simulink model "brain"  (Simulink 7.5)
settings: Solver=FixedStepDiscrete  StartTime=0.0  StopTime=inf  FixedStep=0.2  RelTol=1e-3
values from neighbouring files (symbols this model uses):
  Buoy1_Hue = 0.4    [brainconstants.m]    (also in brainconstants_David.m = 30)
  Buoy1_Saturation = 1.0    (= 1)    [brainconstants.m]    (also in brainconstants_David.m)
  Buoy1_Value = 0.45    [brainconstants.m]    (also in brainconstants_David.m)
  Buoy2_Hue = 0.0    (= 0)    [brainconstants.m]    (also in brainconstants_David.m = 80)
  Buoy2_Saturation = 1.0    (= 1)    [brainconstants.m]    (also in brainconstants_David.m)
  Buoy2_Value = 0.75    [brainconstants.m]    (also in brainconstants_David.m)
  Buoy_Max_Eccentricity = 0.7    [brainconstants.m]    (also in brainconstants_David.m = 1.2)
  Buoy_Max_Extent = 0.9    [brainconstants.m]    (also in brainconstants_David.m)
  Buoy_Min_Eccentricity = 0    [brainconstants.m]    (also in brainconstants_David.m)
  Buoy_Min_Extent = 0.7    [brainconstants.m]    (also in brainconstants_David.m = 0.1)
  Buoy_Strafe = 40    [brainconstants.m]    (also in brainconstants_David.m)
  Cam_Down_Strafe_XPos_Kd = 0.0    (= 0)    [brainconstants.m]    (also in brainconstants_David.m)
  Cam_Down_Strafe_XPos_Ki = 0.0    (= 0)    [brainconstants.m]    (also in brainconstants_David.m)
  Cam_Down_Strafe_XPos_Kp = -1.0    (= -1)    [brainconstants.m]    (also in brainconstants_David.m)
  Cam_Down_Yaw_XPos_Kd = 0.0    (= 0)    [brainconstants.m]    (also in brainconstants_David.m)
  Cam_Down_Yaw_XPos_Ki = 0.0    (= 0)    [brainconstants.m]    (also in brainconstants_David.m)
  Cam_Down_Yaw_XPos_Kp = 0.6    [brainconstants.m]    (also in brainconstants_David.m)
  Cam_Down_YPos_Kd = 0.0    (= 0)    [brainconstants.m]    (also in brainconstants_David.m)
  Cam_Down_YPos_Ki = 0.0    (= 0)    [brainconstants.m]    (also in brainconstants_David.m)
  Cam_Down_YPos_Kp = 0.75    [brainconstants.m]    (also in brainconstants_David.m)
  Cam_Forward_XPosition_Kd = 0.0    (= 0)    [brainconstants.m]    (also in brainconstants_David.m)
  Cam_Forward_XPosition_Ki = 0.0    (= 0)    [brainconstants.m]    (also in brainconstants_David.m)
  Cam_Forward_XPosition_Kp = 0.07    [brainconstants.m]    (also in brainconstants_David.m)
  Cam_Forward_YPosition_Kd = 0.0    (= 0)    [brainconstants.m]    (also in brainconstants_David.m)
  Cam_Forward_YPosition_Ki = 0.0    (= 0)    [brainconstants.m]    (also in brainconstants_David.m)
  Cam_Forward_YPosition_Kp = 0.8    [brainconstants.m]    (also in brainconstants_David.m)
  Depth_Kd = 0.0    (= 0)    [brainconstants.m]    (also in brainconstants_David.m)
  Depth_Ki = 0.0    (= 0)    [brainconstants.m]    (also in brainconstants_David.m)
  Depth_Kp = 75    [brainconstants.m]    (also in brainconstants_David.m)
  Heading_Forward_Velocity = 30    [brainconstants.m]    (also in brainconstants_David.m)
  Heading_Kd = 0.4    [brainconstants.m]    (also in brainconstants_David.m)
  Heading_Ki = 0.0    (= 0)    [brainconstants.m]    (also in brainconstants_David.m)
  Heading_Kp = 0.65    [brainconstants.m]    (also in brainconstants_David.m)
  Hedge_Hue = .4    (= 0.4)    [brainconstants.m]    (also in brainconstants_David.m)
  Hedge_Saturation = 1    [brainconstants.m]    (also in brainconstants_David.m)
  Hedge_Value = .75    (= 0.75)    [brainconstants.m]    (also in brainconstants_David.m)
  Iter_Segment_Thresh = 60    [brainconstants.m]    (also in brainconstants_David.m)
  MissionPlan = [1 1 1 1 1 1 1 1 1 1 1 1 1 0 0 0 0 0 0 0]    [brainconstants.m]    (also in brainconstants_David.m)
  Track_Desired_Depth = 8    [brainconstants.m]    (also in brainconstants_David.m)
  Track_HueHigher = 0.75    [brainconstants.m]    (also in brainconstants_David.m)
  Track_HueLower = 0.4    [brainconstants.m]    (also in brainconstants_David.m)
  Track_Min_Eccentricity = 0.9    [brainconstants.m]    (also in brainconstants_David.m)
  Track_Saturation = 0.75    [brainconstants.m]    (also in brainconstants_David.m)
  Vision_Forward_Velocity = 15    [brainconstants.m]    (also in brainconstants_David.m)
undefined symbols (not defined in the file or in its folder): DiscIntNeverNeededParam, gray, Rec, SDTV, strel, YawRate_Kd, YawRate_Ki, YawRate_Kp
libraries: vipconversions x32, simulink x26, vipgeotforms x9, vipstatistics x9, viptextngfix x7, vipmorphops x6, viptransforms x4, vipsnks x3, vipsrcs x1
(part 4 of 6)

== stateflow chart StateFlow Functions ==
  settings: updateMethod=DISCRETE  sampleTime=0.20
  state StateFlowFunctions [parallel]
    settings: executionOrder=3
    state NotRunning
      entry:
      Left = 0;
      Right = 0;
      Vertical = 0;
      Strafe = 0;
      State = -2;
    state ControlledRC
      entry:
      State = -1;
      exit:
      Left = 0;
      Right = 0;
      Strafe = 0;
      state Compass
        du:
        Vertical = MaintainDepth(CurrentDepth,RC_Depth);
        [Left,Right] = MaintainHeading(RC_Heading,CurrentHeading,RC_ForwardVelocity);
        Strafe = RC_Strafe;
      state IMU
        du:
        Vertical = MaintainDepth(CurrentDepth,RC_Depth);
        [Left, Right,Strafe] = GoStraight(YawRate,PitchAccelB,RC_ForwardVelocity);
      (default) -> Compass
      Compass -> IMU : [RC_Source > 0.5]
      IMU -> Compass : [RC_Source < 0.5]
    state Finish
      entry:
      State = 6;
      Left = 0;
      Right = 0;
      Vertical = 0;
      Strafe = 0;
    state [ChangetoLeft,ChangetoRight] = MaintainHeading(DesiredHeading1, CurrentHeading1, ForwardVelocity1) [function]
    state Buoys
      state RGBout = ShowSegmentedImage(LabMatrix,Ref_Colors) [function]
      state [LabelMatrix,num_colors,Ref_Colors] = IterativeSegmentation(H,S,V) [function]
      state BuoyDone
        en:
        Done = 1;
        Left = 0;
        Right = 0;
        Strafe = 0;
      state FindBuoys
        entry:
        Obstacle = 0;
        OldObstacle = 0;
        CameraPosition = 0;
        BuoyCount = 0;
        DesiredDepth = GetDesiredDepth();
        du:
        [LabelMatrix,num_colors,ref_colors] = IterativeSegmentation(H,S,V);
        RGBout = ShowSegmentedImage(LabelMatrix,ref_colors);
        [Obstacle, RGBout] = LookforBuoys(LabelMatrix,num_colors,RGBout);
        [BuoyCount] = countimages(Obstacle, OldObstacle, BuoyCount);
        Forward = GetBuoyForwardVelocity();
        [Left, Right] = MaintainHeading(DesiredHeading,CurrentHeading,Forward) ;
        [Vertical] = MaintainDepth(CurrentDepth,DesiredDepth);
        OldObstacle = Obstacle;
        exit:
        [BuoyBlobs, num_blobs] = GetBuoyColors(LabelMatrix,ref_colors,num_colors);
        state [Image,RGBout1] = LookforBuoys(LabMatrix,num_colors,RGBin) [function]
        state [L2RBlobs,num_blobs] = GetBuoyColors(LabelMatrix,ref_colors,num_colors) [function]
      state ForwardVel = GetBuoyForwardVelocity [function]
      state ApproachBuoys
        en:
        countarea = 0;
        count2ndarea = 0;
        TurnDirection = 0;
        state ApproachFirstBuoy
          entry:
          [BuoyHue,BuoySaturation,BuoyValue] = GetFirstBuoyStats();
          [FirstDir,SecondDir] = WhichBuoysToApproach(BuoyBlobs,num_blobs);
          du:
          [LabelMatrix,num_colors,ref_colors] = IterativeSegmentation(H,S,V);
          [Area, Right,Left, Vertical, BuoyCentroidX, BuoyCentroidY,BWout] = Buoy(LabelMatrix,ref_colors,num_colors,BuoyHue,BuoySaturation,BuoyValue);
          countarea = countareas(Area, countarea);
          RGBout = ShowSegmentedImage(LabelMatrix,ref_colors);
          state [B_H,B_S,B_V] = GetFirstBuoyStats [function]
          state [FirstD,SecondD] = WhichBuoysToApproach(buoys,num_blobs) [function]
        state [BuoyArea,ChangetoRight,ChangetoLeft,ChangetoVert,CentroidY,CentroidX,BWout1] = Buoy(LabMatrix,Ref_Colors,Num_Colors,B_Hue,B_Sat,B_Value) [function]
        state FindSecondBuoy
          en:
          TurnDirection = -1;
          DesiredHeading = Turn45Degrees(CurrentHeading,TurnDirection);
          DesiredDepth = CurrentDepth;
          [BuoyHue,BuoySaturation,BuoyValue] = GetSecondBuoyStats();
          Image = 0;
          du:
          [Left,Right] = MaintainHeading(DesiredHeading,CurrentHeading,0);
          Vertical = MaintainDepth(CurrentDepth,DesiredDepth);
          Strafe = GetStrafe();
          Strafe = TurnDirection * Strafe;
          [LabelMatrix,num_colors,ref_colors] = IterativeSegmentation(H,S,V);
          [Image, BWout] = SecondBuoy(LabelMatrix,ref_colors,num_colors,BuoyHue,BuoySaturation,BuoyValue);
          RGBout = ShowSegmentedImage(LabelMatrix,ref_colors);
          state [B_H,B_S,B_V] = GetSecondBuoyStats [function]
          state [Image,BWout1] = SecondBuoy(LabMatrix,Ref_Colors,Num_Colors,B_Hue,B_Sat,B_Value) [function]
          state Strafe1 = GetStrafe [function]
        state ApproachSecondBuoy
          entry:
          Strafe = 0;
          du:
          [LabelMatrix,num_colors,ref_colors] = IterativeSegmentation(H,S,V);
          [Area, Right,Left, Vertical, BuoyCentroidX, BuoyCentroidY,BWout] = Buoy(LabelMatrix,ref_colors,num_colors,BuoyHue,BuoySaturation,BuoyValue);
          count2ndarea = countareas(Area, count2ndarea);
          RGBout = ShowSegmentedImage(LabelMatrix,ref_colors);
        (default) -> ApproachFirstBuoy
        ApproachFirstBuoy -> FindSecondBuoy : [countarea>2]
        FindSecondBuoy -> ApproachSecondBuoy : [Image == 1]
      (default) -> FindBuoys
      FindBuoys -> ApproachBuoys : [BuoyCount > 2]
      ApproachBuoys -> BuoyDone : [count2ndarea > 2 || TurnDirection <= -999]
    state ValidationGate
      entry:
      Obstacle = 0;
      OldObstacle = 0;
      count = 0;
      TrackCount = 0;
      CameraPosition = 2;
      state GoThoughGate
        du:
        [Obstacle,BWout] = LookforTrack(H,S);
        [TrackCount] = countimages(Obstacle, OldObstacle, count);
        Forward = GetValidationGateForwardVelocity();
        [Left, Right] = MaintainHeading(DesiredHeading,CurrentHeading,Forward) ;
        [Vertical] = MaintainDepth(CurrentDepth,DesiredDepth);
        OldObstacle = Obstacle;
        count = TrackCount;
      state GateDone
        en:
        Done = 1;
      state [Image,BWout1] = LookforTrack(H,S) [function]
      state ForwardVel=GetValidationGateForwardVelocity [function]
      (default) -> GoThoughGate
      GoThoughGate -> GateDone : [TrackCount > 2]
    state ChangetoVertical = MaintainDepth(CurrentDepth1, DesiredDepth1) [function]
    state Start
      entry:
      OldHeading = 0;
      DesiredHeadingCount = 0;
      BuoyCentroidX = 0;
      BuoyCentroidY = 0;
      CameraPosition = 2;
      Left = 0;
      Right = 0;
      Vertical = 0;
      Strafe = 0;
      state GetHeadings
        du:
        DesiredHeadingCount = InitialHeadingCount(CurrentHeading,OldHeading,DesiredHeadingCount);
        OldHeading = CurrentHeading;
        DesiredDepth = GetDesiredDepth();
        exit:
        DesiredHeading = CurrentHeading;
      state StartFinished
        en:
        Done = 1;
      GetHeadings -> StartFinished : [DesiredHeadingCount >=3]
      (default) -> GetHeadings
    state GetInCorrectState
    state DesiredDepth = GetDesiredDepth [function]
    state FollowOnePath
      entry:
      DesiredDepth = GetDesiredDepth();
      DesiredHeading = CurrentHeading;
      CameraPosition = 2;
      Obstacle = 0;
      HSVImage = MakeHSVImage(H,S,V);
      state OnePath
        state Done
          en:
          Left = 0;
          Right = 0;
          Strafe = 0;
          DesiredHeading = CurrentHeading + HeadingAlongPath;
          Done = 1;
        state PositionOver
          en:
          Error = 500;
          du:
          BWout = HSVSegmentation(H,S);
          [Left,Right,Forward,ErrorX,ErrorY] = CamDown_CenterOver_Yaw(BWout);
          Vertical = MaintainDepth(CurrentDepth,DesiredDepth);
          Left = Left + Forward;
          Right = Right + Forward;
          Error = CalcError(ErrorX,ErrorY);
        state AlignWithPath
          entry:
          HeadingAlongPath = 10;
          Left = 0;
          Right = 0;
          Strafe = 0;
          du:
          [BWout] = HSVSegmentation(H,S);
          [HeadingAlongPath,BWout] = GetHeadings(BWout);
          [Left,Right,Forward,ErrorY,ErrorX] = CamDown_CenterOver_Yaw(BWout);
          Vertical = MaintainDepth(CurrentDepth,DesiredDepth);
          Strafe = Align(HeadingAlongPath);
          state Strafe = Align(HeadingAlong) [function]
          state [HeadingAlongPath1,BWout1] = GetHeadings(BW) [function]
        state BW1 = HSVSegmentation(H,S) [function]
        state [Strafe1,Forward1,ErrorX1,ErrorY1,BWout1] = CenterOver_Strafe(BW) [function]
        state [Left1,Right1,Forward1,ErrorY1,ErrorX1] = CamDown_CenterOver_Yaw(BW) [function]
        PositionOver -> AlignWithPath : [Error < 10]
        AlignWithPath -> StateFlowFunctions.FollowOnePath.OnePath.Done : [abs(HeadingAlongPath) <= 4]
        (default) -> PositionOver
      state RecognizePath
        du:
        [Obstacle,BWout] = LookforTrack(H,S);
        state TurnRight
          du:
          DesiredHeading = CurrentHeading + 15;
          [Left,Right] = MaintainHeading(DesiredHeading,CurrentHeading,0);
          [Vertical] = MaintainDepth(CurrentDepth,DesiredDepth);
        state TurnLeft
          du:
          DesiredHeading = CurrentHeading - 15;
          [Left,Right] = MaintainHeading(DesiredHeading,CurrentHeading,0);
          [Vertical] = MaintainDepth(CurrentDepth,DesiredDepth);
        state [Image,BWout1] = LookforTrack(H,S) [function]
        (default) -> TurnLeft
        TurnLeft -> TurnRight : after(1,sec)
        TurnRight -> TurnLeft : after(1,sec)
      state HSVImage1 = MakeHSVImage(H1,S1,V1) [function]
      (default) -> RecognizePath
      RecognizePath -> OnePath : [Obstacle == 1]
    state JumpHedge
      entry:
      Area = 1000;
      Left = 0;
      Right = 0;
      Strafe = 0;
      Done = 0;
      Image = 0;
      state ApproachHedge
        du:
        [LabelMatrix,num_colors,ref_colors] = IterativeSegmentation(H,S,V);
        BWout = IndividualSegmentation(LabelMatrix,ref_colors,num_colors,H_Hue,H_Sat,H_Value);
        [Left,Right,Vertical,BWout] = CameraForward_CenterOnBlobYaw(BWout,Forward);
        Area = GetArea(BWout);
        RGBout = ShowSegmentedImage(LabelMatrix,ref_colors);
        state AreaBiggestBlob = GetArea(BW) [function]
      state IncreaseAxisRatio
        exit:
        Strafe = 0;
        Left = 0;
        Right = 0;
        state Move
          du:
          [LabelMatrix,num_colors,ref_colors] = IterativeSegmentation(H,S,V);
          BWout = IndividualSegmentation(LabelMatrix,ref_colors,num_colors,H_Hue,H_Sat,H_Value);
          [Right,Left,Vertical] = CameraForward_CenterOnBlobYaw(BWout,0);
          Strafe = 40*StrafeDir;
          RGBout = ShowSegmentedImage(LabelMatrix,ref_colors);
          exit:
          Strafe = 0;
          Left = 0;
          Right = 0;
        state CheckAxisRatio
          en:
          NewAxisRatio = GetAxisRatio(BWout);
        (default) -> StateFlowFunctions.JumpHedge.IncreaseAxisRatio.Move
        StateFlowFunctions.JumpHedge.IncreaseAxisRatio.Move -> CheckAxisRatio : after(1,sec)
        CheckAxisRatio -> StateFlowFunctions.JumpHedge.IncreaseAxisRatio.Move
      state GetInitialDirection
        state GetMajorAxis
          entry:
          MoveOn = 0;
          OldAxisRatio = 0.5;
          StrafeDir = 1;
          [LabelMatrix,num_colors,ref_colors] = IterativeSegmentation(H,S,V);
          BWout = IndividualSegmentation(LabelMatrix,ref_colors,num_colors,H_Hue,H_Sat,H_Value);
          OldAxisRatio = GetAxisRatio(BWout);
          RGBout = ShowSegmentedImage(LabelMatrix,ref_colors);
        state Move
          du:
          [LabelMatrix,num_colors,ref_colors] = IterativeSegmentation(H,S,V);
          BWout = IndividualSegmentation(LabelMatrix,ref_colors,num_colors,H_Hue,H_Sat,H_Value);
          [Right,Left,Vertical] = CameraForward_CenterOnBlobYaw(BWout,0);
          Strafe = 40*StrafeDir;
          RGBout = ShowSegmentedImage(LabelMatrix,ref_colors);
          exit:
          Strafe = 0;
        state CompareAxisRatio
          entry:
          [LabelMatrix,num_colors,ref_colors] = IterativeSegmentation(H,S,V);
          BWout = IndividualSegmentation(LabelMatrix,ref_colors,num_colors,H_Hue,H_Sat,H_Value);
          NewAxisRatio = GetAxisRatio(BWout);
          AxisDifference = NewAxisRatio - OldAxisRatio;
          StrafeDir = GetStrafeDirection(AxisDifference);
          MoveOn = 1;
          RGBout = ShowSegmentedImage(LabelMatrix,ref_colors);
        (default) -> GetMajorAxis
        StateFlowFunctions.JumpHedge.GetInitialDirection.Move -> CompareAxisRatio : after(2,sec)
        GetMajorAxis -> StateFlowFunctions.JumpHedge.GetInitialDirection.Move
      state RecognizeHedge
        en:
        [H_Hue,H_Sat,H_Value] = GetHedgeValues();
        Forward = GetForwardVelocity();
        du:
        [LabelMatrix,num_colors,ref_colors] = IterativeSegmentation(H,S,V);
        BWout = IndividualSegmentation(LabelMatrix,ref_colors,num_colors,H_Hue,H_Sat,H_Value);
        [Left,Right] = MaintainHeading(DesiredHeading,CurrentHeading,Forward);
        [Vertical] = MaintainDepth(CurrentDepth,DesiredDepth);
        [Image,BWout] = LookForHedge(BWout);
        RGBout = ShowSegmentedImage(LabelMatrix,ref_colors);
        state [Image1,BWout1] = LookForHedge(BW) [function]
        state [H_hue,H_sat,H_val] = GetHedgeValues [function]
      state BW = IndividualSegmentation(LabMatrix,Ref_Colors,Num_Colors,B_Hue,B_Sat,B_Value) [function]
      state GoThroughHedge
        en:
        DesiredHeading = CurrentHeading;
        DesiredDepth = CurrentDepth - 2;
        Strafe = 0;
        du:
        [LabelMatrix,num_colors,ref_colors] = IterativeSegmentation(H,S,V);
        BWout = IndividualSegmentation(LabelMatrix,ref_colors,num_colors,H_Hue,H_Sat,H_Value);
        [Left,Right] = MaintainHeading(DesiredHeading,CurrentHeading,Forward);
        [Vertical] = MaintainDepth(CurrentDepth,DesiredDepth);
        RGBout = ShowSegmentedImage(LabelMatrix,ref_colors);
      state RGBout = ShowSegmentedImage(LabMatrix,Ref_Colors) [function]
      state [LabelMatrix,num_colors,Ref_Colors] = IterativeSegmentation(H,S,V) [function]
      state Finished
        en:
        Left = 0;
        Right = 0;
        Strafe = 0;
        Done = 1;
      state [ChangetoLeft,ChangetoRight,ChangetoVert,BWout1] = CameraForward_CenterOnBlobYaw(BW,ForwardVelocity) [function]
      state AxisRatio = GetAxisRatio(BW) [function]
      state ForwardVel=GetForwardVelocity [function]
      GetInitialDirection -> ApproachHedge [order 1] : [OldAxisRatio > 1 || NewAxisRatio > 1]
      (default) -> RecognizeHedge
      RecognizeHedge -> GetInitialDirection : [Image == 1]
      IncreaseAxisRatio -> ApproachHedge : [NewAxisRatio > 1]
      GetInitialDirection -> IncreaseAxisRatio [order 2] : [MoveOn == 1]
      ApproachHedge -> GoThroughHedge : [Area > 4000]
      GoThroughHedge -> StateFlowFunctions.JumpHedge.Finished : after(5,sec)
    state DropMechanism
      en:
      Done = 1;
    state LocatePinger
      en:
      Done = 1;
      MoveOn = 0;
      OldDesiredHeading = DesiredHeading;
      exit:
      Left = 0;
      Right = 0;
      Vertical = 0;
      state Finished
        en:
        Done = changemeasure(DesiredHeading,OldDesiredHeading);
      state GetPingerHeading
        en:
        Left = 0;
        Right = 0;
        OldDesiredHeading = DesiredHeading;
        du:
        Vertical = MaintainDepth(CurrentDepth,DesiredDepth);
        state FirstDirections
          en:
          [Heading1, Heading2] = GetHeadings();
        state SecondDirections
          en:
          Left = 0;
          Right = 0;
          [Heading3,Heading4] = GetHeadings();
        state Turn30Degrees
          en:
          DesiredHeading = Turn30(CurrentHeading);
          du:
          [Left,Right] = MaintainHeading(DesiredHeading,CurrentDepth,0);
        state GetActualDirection
          en:
          DesiredHeading = ProperHeading(Heading1,Heading2,Heading3,Heading4);
        state GoToNext
          MoveOn = 1;
        state [Heading11,Heading22] = GetHeadings [function]
        FirstDirections -> Turn30Degrees
        Turn30Degrees -> SecondDirections : [abs(CurrentHeading-DesiredHeading) < 5]
        SecondDirections -> GetActualDirection
        GetActualDirection -> FirstDirections [order 1] : [DesiredHeading == -1]
        GetActualDirection -> GoToNext [order 2] : [DesiredHeading ~= -1]
        (default) -> FirstDirections
      state Move
        du:
        [Left,Right] = MaintainHeading(DesiredHeading,CurrentHeading,Forward);
        Vertical = MaintainDepth(CurrentDepth,DesiredDepth);
      GetPingerHeading -> StateFlowFunctions.LocatePinger.Finished : [MoveOn ~= 0]
      StateFlowFunctions.LocatePinger.Move -> GetPingerHeading : after(3,sec)
      StateFlowFunctions.LocatePinger.Finished -> StateFlowFunctions.LocatePinger.Move
      (default) -> GetPingerHeading
    state Breach
      en:
      Left = 0;
      Right = 0;
      Vertical = -127;
      Strafe = 0;
      exit:
      Vertical = 0;
      state GoUpNCheck
      state MakeSure
      state Done
        Done = 1;
      (default) -> GoUpNCheck
      GoUpNCheck -> MakeSure : [CurrentDepth < 0.5]
      MakeSure -> StateFlowFunctions.Breach.Done : after(3,sec)
    state [ChangetoLeft1,ChangetoRight1,Strafe1] = GoStraight(YawRate,ForwardVelocity1,Y_Accel) [function]
    StateFlowFunctions.Finish -> GetInCorrectState : [OperationalState ~= 9]
    (default) -> GetInCorrectState
    StateFlowFunctions.NotRunning -> GetInCorrectState : [OperationalState ~= -2]
    GetInCorrectState -> StateFlowFunctions.NotRunning [order 1] : [OperationalState == -2]
    GetInCorrectState -> StateFlowFunctions.ControlledRC [order 3] : [OperationalState == -1]
    StateFlowFunctions.ControlledRC -> GetInCorrectState : [OperationalState ~= -1]
    StateFlowFunctions.Start -> GetInCorrectState : [OperationalState ~= 1]
    GetInCorrectState -> StateFlowFunctions.Start [order 4] : [OperationalState == 1]
    GetInCorrectState -> StateFlowFunctions.ValidationGate [order 5] : [OperationalState == 2]
    StateFlowFunctions.ValidationGate -> GetInCorrectState : [OperationalState ~= 2]
    FollowOnePath -> GetInCorrectState : [OperationalState ~= 3]
    GetInCorrectState -> FollowOnePath [order 7] : [OperationalState == 3]
    Buoys -> GetInCorrectState : [OperationalState ~= 4]
    GetInCorrectState -> Buoys [order 8] : [OperationalState == 4]
    GetInCorrectState -> StateFlowFunctions.Finish [order 6] : [OperationalState == 9]
    GetInCorrectState -> JumpHedge [order 2] : [OperationalState == 5]
    JumpHedge -> GetInCorrectState : [OperationalState ~= 5]
    StateFlowFunctions.DropMechanism -> GetInCorrectState : [OperationalState ~= 6]
    GetInCorrectState -> StateFlowFunctions.DropMechanism [order 9] : [OperationalState == 6]
    GetInCorrectState -> StateFlowFunctions.LocatePinger [order 10] : [OperationalState == 7]
    StateFlowFunctions.LocatePinger -> GetInCorrectState : [OperationalState ~= 7]
    GetInCorrectState -> StateFlowFunctions.Breach [order 11] : [OperationalState == 8]
    StateFlowFunctions.Breach -> GetInCorrectState : [OperationalState ~=8]
  state StateManagement [parallel]
    settings: executionOrder=2
    state NotRunning
      en:
      Done = 0;
      du:
      OperationalState = -2;
    state Running
      state Autonomous
        state Buoy
          en:
          State = 4;
          Done = Perform(State);
          du:
          OperationalState = 4;
        state ValidationGate
          en:
          State = 2;
          Done = Perform(State);
          du:
          OperationalState = 2;
        state Finish
          en:
          State = 13;
          Done = Perform(State);
          du:
          OperationalState = 9;
        state FollowOnePath1
          en:
          State = 3;
          Done = Perform(State);
          du:
          OperationalState = 3;
        state ChooseState
          en:
          Done = 0;
        state FollowOnePath2
          en:
          State = 5;
          Done = Perform(State);
          du:
          OperationalState = 3;
        state Start
          en:
          State = 1;
          Done = Perform(State);
          du:
          OperationalState = 1;
        state Hedge1
          en:
          State = 6;
          Done = Perform(State);
          du:
          OperationalState = 5;
        state FollowOnePath3
          en:
          State = 7;
          Done = Perform(State);
          du:
          OperationalState = 3;
        state DropMechanism
          en:
          State = 8;
          Done = Perform(State);
          du:
          OperationalState = 6;
        state FollowOnePath4
          en:
          State = 9;
          Done = Perform(State);
          du:
          OperationalState = 3;
        state Hedge2
          en:
          State = 10;
          Done = Perform(State);
          du:
          OperationalState = 5;
        state LocatePinger
          en:
          State = 11;
          Done = Perform(State);
          du:
          OperationalState = 7;
        state Breach
          en:
          State = 12;
          Done = Perform(State);
          du:
          OperationalState = 8;
        state Done1 = Perform(State1) [function]
        FollowOnePath1 -> ChooseState [order 2] : [DesiredState ~= 3 && DesiredState ~= 0]
        ChooseState -> FollowOnePath1 [order 6] : [DesiredState == 3]
        StateManagement.Running.Autonomous.ValidationGate -> ChooseState [order 1] : [DesiredState ~= 2 && DesiredState ~= 0]
        ChooseState -> StateManagement.Running.Autonomous.ValidationGate [order 3] : [DesiredState == 2]
        FollowOnePath2 -> ChooseState [order 1] : [DesiredState ~= 5 && DesiredState ~= 0]
        ChooseState -> FollowOnePath2 [order 7] : [DesiredState == 5]
        FollowOnePath1 -> Buoy [order 1] : [Done ~= 0 && DesiredState == 0]
        Buoy -> FollowOnePath2 [order 1] : [Done ~= 0 && DesiredState == 0]
        StateManagement.Running.Autonomous.Breach -> StateManagement.Running.Autonomous.Finish [order 2] : [Done ~= 0 && DesiredState == 0]
        StateManagement.Running.Autonomous.Start -> StateManagement.Running.Autonomous.ValidationGate [order 1] : [Done ~= 0 && DesiredState == 0]
        StateManagement.Running.Autonomous.ValidationGate -> FollowOnePath1 [order 2] : [Done ~=0 && DesiredState == 0]
        (default) -> StateManagement.Running.Autonomous.Start
        ChooseState -> Buoy [order 4] : [DesiredState == 4]
        StateManagement.Running.Autonomous.Finish -> ChooseState : [DesiredState ~= 7 && DesiredState ~= 7]
        StateManagement.Running.Autonomous.Start -> ChooseState [order 2] : [DesiredState ~= 1 && DesiredState ~= 0]
        ChooseState -> StateManagement.Running.Autonomous.Start [order 1] : [DesiredState == 1 || DesiredState == 0]
        Buoy -> ChooseState [order 2] : [DesiredState ~= 4 && DesiredState ~= 0]
        FollowOnePath2 -> Hedge1 [order 2] : [Done ~= 0 && DesiredState == 0]
        Hedge1 -> ChooseState [order 1] : [DesiredState ~= 6 && DesiredState ~= 0]
        ChooseState -> Hedge1 [order 2] : [DesiredState == 6]
        Hedge1 -> FollowOnePath3 [order 2] : [Done ~= 0 && DesiredState == 0]
        FollowOnePath3 -> ChooseState [order 1] : [DesiredState ~= 7 && DesiredState ~= 0]
        ChooseState -> FollowOnePath3 [order 8] : [DesiredState == 7]
        FollowOnePath3 -> StateManagement.Running.Autonomous.DropMechanism [order 2] : [Done ~= 0 && DesiredState == 0]
        StateManagement.Running.Autonomous.DropMechanism -> ChooseState [order 1] : [DesiredState ~= 8 && DesiredState ~= 0]
        ChooseState -> StateManagement.Running.Autonomous.DropMechanism [order 9] : [DesiredState == 8]
        FollowOnePath4 -> ChooseState [order 1] : [DesiredState ~= 0 && DesiredState ~= 9]
        ChooseState -> FollowOnePath4 [order 10] : [DesiredState == 9]
        Hedge2 -> ChooseState [order 1] : [DesiredState ~= 0 && DesiredState ~= 10]
        ChooseState -> Hedge2 [order 11] : [DesiredState == 10]
        FollowOnePath4 -> Hedge2 [order 2] : [Done ~= 0 && DesiredState == 0]
        StateManagement.Running.Autonomous.LocatePinger -> ChooseState [order 1] : [DesiredState ~= 0 && DesiredState ~= 11]
        ChooseState -> StateManagement.Running.Autonomous.LocatePinger [order 5] : [DesiredState == 11]
        Hedge2 -> StateManagement.Running.Autonomous.LocatePinger [order 2] : [Done ~= 0 && DesiredState == 0]
        StateManagement.Running.Autonomous.DropMechanism -> FollowOnePath4 [order 2] : [Done ~= 0 && DesiredState == 0]
        StateManagement.Running.Autonomous.Breach -> ChooseState [order 1] : [DesiredState ~= 0 && DesiredState ~= 12]
        ChooseState -> StateManagement.Running.Autonomous.Breach [order 12] : [DesiredState == 12]
        StateManagement.Running.Autonomous.LocatePinger -> StateManagement.Running.Autonomous.Breach [order 2] : [Done ~= 0 && DesiredState == 0]
      state ControlledRC
        du:
        OperationalState = -1;
      StateManagement.Running.ControlledRC -> Autonomous : [RC == 0]
      Autonomous -> StateManagement.Running.ControlledRC : [RC == 1]
      (default) -> Autonomous
    Running -> StateManagement.NotRunning : [Status ~= 1]
    (default) -> StateManagement.NotRunning
    StateManagement.NotRunning -> Running : [Status == 1]
  state StateEstimator [parallel]
    du:
    Tare1 = Tare;
    settings: executionOrder=1
    state CalcTare
      en:
      TareDone = 0;
      state PerformTare
        en:
        DeltaT1 = CheckDeltaT(DeltaT);
        Yaw1 = CurrentHeading - TarYaw;
        YawRate1 = YawRate - TarYawRate;
        Pitch1 = PitchEuler - TarPitch;
        PitchRate1 = PitchRate - TarPitchRate;
        Roll1 = RollEuler - TarRoll;
        RollRate1 = RollRate - TarRollRate;
        YawRate_Model = AUV_Yaw_Model(Left,Right,OldYawRate,DeltaT1);
        YawRate_Out = combinevalues(YawRate_Model,YawRate1,0.7,0.48);
        OldYawRate = YawRate_Out;
        [Yaw_IMU, Pitch_IMU, Roll_IMU] = Integrate3(YawRate_Out,PitchRate1,RollRate1,OldYaw,OldPitch,OldRoll,DeltaT1);
        Yaw = Yaw_IMU;
        OldYaw = Yaw;
        Pitch = combinevalues(Pitch_IMU,Pitch1,0.75,1);
        OldPitch = Pitch;
        Roll = combinevalues(Roll_IMU,Roll1,0.75,1);
        [Yaw_IMU, Pitch_IMU, Roll_IMU] = Integrate3(YawRate,PitchRate,RollRate,OldYaw,OldPitch,OldRoll,DeltaT1);
        Yaw = combinevalues(Yaw_IMU,CurrentHeading,.75,1);
        OldYaw = Yaw;
        Pitch = combinevalues(Pitch_IMU,PitchEuler,.75,1);
        OldPitch = Pitch;
        Roll = combinevalues(Roll_IMU,RollEuler,.75,1);
        OldRoll = Roll;
        TRA = RollAccelB;
        TPA = PitchAccelB;
        TYA = YawAccelB;
      state Stop
        en:
        Left = 0;
        Right = 0;
        Strafe = 0;
        Vertical = 0;
        stepcount = 0;
        TarYaw = CurrentHeading;
        TarYawRate = YawRate;
        TarPitch = PitchEuler;
        TarPitchRate = PitchRate;
        TarRoll = RollEuler;
        TarRollRate = RollRate;
        OldYaw = 0;
        OldYawRate = 0;
        OldPitch = 0;
        OldRoll = 0;
        OldXVel = 0;
        OldYVel = 0;
        OldZVel = 0;
        OldX = 0;
        OldY = 0;
        OldZ = 0;
        du:
        stepcount = stepcount + 1;
      state Next
        en:
        TareDone = 1;
      (default) -> Stop
      Stop -> PerformTare : [stepcount >= 10]
      PerformTare -> Next
    state CalcIMUInfo
      du:
      DeltaT1 = CheckDeltaT(DeltaT);
      YawRate1 = YawRate - TarYawRate;
      Pitch1 = PitchEuler - TarPitch;
      PitchRate1 = PitchRate - TarPitchRate;
      Roll1 = RollEuler - TarRoll;
      RollRate1 = RollRate - TarRollRate;
      YawRate_Model = AUV_Yaw_Model(Left,Right,OldYawRate,DeltaT1);
      YawRate_Out = combinevalues(YawRate_Model,YawRate1,0.7,0.48);
      OldYawRate = YawRate_Out;
      PitchRate_Out = PitchRate1;
      RollRate_Out = RollRate1;
      [Yaw_IMU, Pitch_IMU, Roll_IMU] = Integrate3(YawRate_Out,PitchRate1,RollRate1,OldYaw,OldPitch,OldRoll,DeltaT1);
      Yaw = Yaw_IMU;
      OldYaw = Yaw;
      Pitch = combinevalues(Pitch_IMU,Pitch1,0.75,1);
      OldPitch = Pitch;
      Roll = combinevalues(Roll_IMU,Roll1,0.75,1);
      OldRoll = Roll;
      Roll_AccelB = (RollAccelB - TRA)/0.3048;
      Pitch_AccelB = (PitchAccelB - TPA)/0.3048;
      Yaw_AccelB = (YawAccelB - TYA)/0.3048;
      [Roll_Accel,Pitch_Accel,Yaw_Accel] = GoToEarthCFrame(Roll_AccelB,Pitch_AccelB,Yaw_AccelB,Yaw,Pitch,Roll);
      [XVel,YVel,ZVel] = Integrate3(Roll_Accel,Pitch_Accel,Yaw_Accel,OldXVel,OldYVel,OldZVel,DeltaT1);
      OldXVel = XVel;
      OldYVel = YVel;
      OldZVel = ZVel;
      [X,Y,Z] = Integrate3(XVel,YVel,ZVel,OldX,OldY,OldZ,DeltaT1);
    (default) -> CalcTare
    CalcIMUInfo -> CalcTare : [Tare1 > 0.5]
    CalcTare -> CalcIMUInfo : [TareDone > 0.5]
  data: CHeading function_input double; TurnD function_input double; DHeading function_output double; FirstD function_input double; SecondD function_input double; TurnD function_output double; B_H function_output double; B_S function_output double; B_V function_output double; LabMatrix function_input double; Ref_Colors function_input double; BuoyArea function_output double; ChangetoRight function_output double; ChangetoLeft function_output double; ChangetoVert function_output double; CentroidY function_output double; CentroidX function_output double; BWout1 function_output double; Num_Colors function_input double; B_Hue function_input double; B_Sat function_input double; B_Value function_input double; LabMatrix function_input double; num_colors function_input double; Image function_output double; RGBin function_input double; RGBout1 function_output double; Size function_input double; count1 function_input double; count2 function_output double; LabMatrix function_input double; Ref_Colors function_input double; RGBout function_output double; H function_input double; S function_input double; V function_input double; LabelMatrix function_output double; num_colors function_output double; Ref_Colors function_output double; LabelMatrix function_input double; ref_colors function_input double; num_colors function_input double; L2RBlobs function_output double; num_blobs function_output double; DesiredHeading1 function_input double; CurrentHeading1 function_input double; ChangetoLeft function_output double; ChangetoRight function_output double; ForwardVelocity1 function_input double; B_H function_output double; B_S function_output double; B_V function_output double; Image function_output double; LabMatrix function_input double; Ref_Colors function_input double; BWout1 function_output double; Num_Colors function_input double; B_Hue function_input double; B_Sat function_input double; B_Value function_input double; ForwardVel function_output double; buoys function_input double; num_blobs function_input double; FirstD function_output double; SecondD function_output double; Image1 function_input double; OldImage function_input double; count1 function_input double; count2 function_output double; Strafe1 function_output double; Image function_input double; OldImage function_input double; count1 function_input double; count2 function_output double; Image function_output double; H function_input double; S function_input double; BWout1 function_output double; ForwardVel function_output double; CurrentDepth1 function_input double; DesiredDepth1 function_input double; ChangetoVertical function_output double; CurrentHeading1 function_input double; DesiredHeadingCount1 function_output double; OldHeading1 function_input double; count1 function_input double; DesiredDepth function_output double; ErrorX1 function_input double; ErrorY1 function_input double; Error1 function_output double; HeadingAlong function_input double; Strafe function_output double; BW function_input double; HeadingAlongPath1 function_output double; BWout1 function_output double; H function_input double; BW1 function_output double; S function_input double; BW function_input double; Strafe1 function_output double; Forward1 function_output double; ErrorX1 function_output double; ErrorY1 function_output double; BWout1 function_output double; Image function_output double; H function_input double; S function_input double; BWout1 function_output double; H1 function_input double; S1 function_input double; V1 function_input double; HSVImage1 function_output double; AreaBiggestBlob function_output double; BW function_input double; AxisDif function_input double; StrafeDir1 function_output double; BW function_input double; Image1 function_output double; BWout1 function_output double; H_hue function_output double; H_sat function_output double; H_val function_output double; LabMatrix function_input double; Ref_Colors function_input double; Num_Colors function_input double; B_Hue function_input double; B_Sat function_input double; B_Value function_input double; BW function_output double; LabMatrix function_input double; Ref_Colors function_input double; RGBout function_output double; H function_input double; S function_input double; V function_input double; LabelMatrix function_output double; num_colors function_output double; Ref_Colors function_output double; ChangetoLeft function_output double; ChangetoRight function_output double; ChangetoVert function_output double; BW function_input double; ForwardVelocity function_input double; BWout1 function_output double; BW function_input double; AxisRatio function_output double; AxisDif function_input double; StrafeDirection function_input double; Strafeout function_output double; ForwardVel function_output double; CurrentDepth1 function_input double; Done1 function_output double; signal1 function_input double; DesiredHeading1 function_output double; DesiredHeading1 function_input double; OldDesiredHeading1 function_input double; finished function_output double; CurrentHeading1 function_input double; heading function_output double; Heading11 function_input double; Heading22 function_input double; Heading33 function_input double; Heading44 function_input double; heading function_output double; Heading11 function_output double; Heading22 function_output double; State1 function_input double; Done1 function_output double; BW function_input double; Left1 function_output double; Right1 function_output double; Forward1 function_output double; ErrorY1 function_output double; ErrorX1 function_output double; YawRate function_input double; ForwardVelocity1 function_input double; ChangetoLeft1 function_output double; ChangetoRight1 function_output double; Y_Accel function_input double; Strafe1 function_output double; r function_input double; yaw1 function_input double; value function_output double; deltaT function_input double; Yr function_input double; Pr function_input double; Rr function_input double; OY function_input double; OP function_input double; OR function_input double; Y1 function_output double; P1 function_output double; R1 function_output double; deltaT function_input double; delta function_input double; delta1 function_output double; RAccB function_input double; PAccB function_input double; YAccB function_input double; R_Acc function_output double; P_Acc function_output double; Y_Acc function_output double; y function_input double; p function_input double; r function_input double; r_m function_input double; r1 function_input double; r function_output double; e1 function_input double; e2 function_input double; L1 function_input double; R1 function_input double; r_0 function_input double; r function_output double; deltaT function_input double; Left output int8 size=1; CurrentDepth input double size=1; CurrentHeading input double size=1; Right output int8 size=1; Strafe output int8; Vertical output int8 size=1; DesiredDepth output double; count local double; Obstacle local boolean size=1; OldObstacle local boolean; DesiredHeading output double; Area local int32; countarea local double; CameraPosition output int8 size=1; H input single size=[120 160]; S input single size=[120 160]; V input single size=[120 160]; BuoyCentroidX output double; BuoyCentroidY output double; DesiredHeadingCount local double; OldHeading local double; TrackCount local double; BuoyCount local double; State output int8 size=1; Status input int8 size=1; DesiredState input int8; HSVImage local double size=[120 160 3]; HeadingAlongPath local double; Done local double; RC_Heading input double; RC_ForwardVelocity input double; RC_Strafe input double; RC_Depth input double; RC input boolean; Error local double; ErrorX local double; ErrorY local double; Forward local double; BWout output double size=[120 160]; OperationalState local int8; BuoyHue local double; BuoySaturation local double; BuoyValue local double; FirstDir local double; Image local double; LabelMatrix local double size=[120 160]; RGBout output double size=[120 160 3]; SecondDir local double; TurnDirection local double; count2ndarea local double; num_colors local double; ref_colors local double size=[50 3]; num_blobs local double; BuoyBlobs local double size=[50 4]; AxisDifference local double; H_Hue local double; H_Sat local double; H_Value local double; MoveOn local double; NewAxisRatio local double; OldAxisRatio local double; StrafeDir local double; Heading1 local double; Heading2 local double; Heading3 local double; Heading4 local double; OldDesiredHeading local double; YawRate input double; PitchRate input double; PitchAccelB input double; PitchEuler input double; RollRate input double; RollAccelB input double; RollEuler input double; YawAccelB input double; Tare input double; DeltaT input double; OldPitch local double; OldRoll local double; OldX local double; OldXVel local double; OldY local double; OldYVel local double; OldYaw local double; OldYawRate local double; OldZ local double; OldZVel local double; Pitch_IMU local double; Roll_IMU local double; TPA local double; TRA local double; TYA local double; YawRate_Model local double; Yaw_IMU local double; Tare1 local double; stepcount local double; Pitch output double; Roll output double; Yaw output double; X output double; Y output double; Z output double; XVel output double; YVel output double; ZVel output double; Pitch_Accel output double; Roll_Accel output double; Yaw_Accel output double; PitchRate_Out output double; RollRate_Out output double; YawRate_Out output double; RC_Source input double; DeltaT1 local double; Pitch1 local double; PitchRate1 local double; Roll1 local double; RollRate1 local double; TarPitch local double; TarPitchRate local double; TarRoll local double; TarRollRate local double; TarYaw local double; TarYawRate local double; Yaw1 local double; YawRate1 local double; Pitch_AccelB local double; Roll_AccelB local double; TareDone local double; Yaw_AccelB local double
  function DHeading = Turn45Degrees(CHeading,TurnD):
    | function DHeading = Turn45Degrees(CHeading,TurnD)
    | % This function changes the current heading by 45 degrees in the correct
    | % direction to see the next buoy
    | 
    | DHeading = CHeading + TurnD*45;
    | 
    | if(DHeading > 360)
    |     DHeading = DHeading - 360;
    | elseif(DHeading < 0)
    |     DHeading = DHeading + 360;
    | end
    | 
    | return
  function TurnD = GetDirectionToLook(FirstD,SecondD):
    | function TurnD = GetDirectionToLook(FirstD,SecondD)
    | % Determine which direction the AUV needs to turn to see the next buoy
    | % -1 is left, 1 is right, -999 is for a single buoy attempt
    | 
    | % FirstD, SecondD are 1,2,3 - left,middle,right
    | TurnD = SecondD - FirstD;
    | 
    | if(TurnD ~= 0)
    |     TurnD = TurnD / abs(TurnD);
    | else
    |     TurnD = -999;
    | end
    | 
    | return
  function count2 = countareas(Size, count1):
    | function count2 = countareas(Size, count1)
    | % This function acts to count the number of consecutive times a particular
    | % area is recognized by the recognition software
    | 
    | count2 = count1;
    | if(Size > 16000)
    |     count2 = count2 + 1;
    | else
    |     count2 = 0;
    | end
  function count2 = countimages(Image1, OldImage, count1):
    | function count2 = countimages(Image1, OldImage, count1)
    | % This function acts to count the number of consecutive times a particular
    | % image is recognized by the recognition software
    | 
    | count2 = count1;
    | if(Image1 == 1)
    |     count2 = count2 + 1;
    | else
    |     count2 = 0;
    | end
  function count2 = countimages(Image, OldImage, count1):
    | function count2 = countimages(Image, OldImage, count1)
    | % This function acts to count the number of consecutive times a particular
    | % image is recognized by the recognition software
    | 
    | count2 = count1;
    | if(Image ~= 0 && Image == OldImage)
    |     count2 = count2 + 1;
    | else
    |     count2 = 0;
    | end
  function DesiredHeadingCount1 = InitialHeadingCount(CurrentHeading1,OldHeading1,count1):
    | function DesiredHeadingCount1 = InitialHeadingCount(CurrentHeading1,OldHeading1,count1)
    | 
    | tolerance = 2;
    | 
    | if(CurrentHeading1 > OldHeading1 - tolerance && CurrentHeading1 < OldHeading1 + tolerance)
    |     count1 = count1 + 1;
    | else
    |     count1 = 0;
    | end
    | DesiredHeadingCount1 = count1;
  function Error1 = CalcError(ErrorX1,ErrorY1):
    | function Error1 = CalcError(ErrorX1,ErrorY1)
    | % This function calculates the error between the center of the screen and 
    | % the centroid of the orange/red blob
    | 
    | Error1 = abs(ErrorX1) + abs(ErrorY1);
    | 
    | return
  function StrafeDir1 = GetStrafeDirection(AxisDif):
    | function StrafeDir1 = GetStrafeDirection(AxisDif)
    | % This function determines the direction the AUV should be strafing based
    | % on the initial major axis length change when strafing right
    | 
    | if(AxisDif < 0)
    |     StrafeDir1 = -1;
    | else
    |     StrafeDir1 = 1;
    | end
    | 
    | % StrafeDir = -1 corresponds to strafing left
    | % StrafeDir = 1 corresponds to strafing right
    | 
    | return
  function Strafeout = CalcStrafe(AxisDif,StrafeDirection):
    | function Strafeout = CalcStrafe(AxisDif,StrafeDirection)
    | % This function determines the current command to the strafing thruster
    | 
    | Kp = 4;
    | 
    | Strafeout = Kp * AxisDif * StrafeDirection;
    | 
    | return
  function Done1 = BreachDone(CurrentDepth1):
    | function Done1 = BreachDone(CurrentDepth1)
    | % This function determines if the vehicle has breached
    | 
    | if(CurrentDepth1 < 0.5)
    |     Done1 = 1;
    | else
    |     Done1 = 0;
    | end
    | 
    | return
  function DesiredHeading1=CalcPingerDirection(signal1):
    | function DesiredHeading1=CalcPingerDirection(signal1)
    | % This function determines the direction to the pinger given a signal from
    | % it
    | 
    | DesiredHeading1 = 0;
    | 
    | return
  function finished = changemeasure(DesiredHeading1,OldDesiredHeading1):
    | function finished = changemeasure(DesiredHeading1,OldDesiredHeading1)
    | % This function determines if the heading changes a large enough amount to 
    | % imply that the auv is above the pinger
    | 
    | finished = 0;
    | 
    | heading_change = DesiredHeading1 - OldDesiredHeading1;
    | 
    | if(abs(heading_change) > 60)
    |     finished = 1;
    | end
    | 
    | return
  function heading = Turn30(CurrentHeading1):
    | function heading = Turn30(CurrentHeading1)
    | % This function determines the heading to turn 30 degrees to the right
    | 
    | heading = CurrentHeading1 + 30;
    | 
    | if(heading >= 360)
    |     heading = heading - 360;
    | end
    | 
    | return
  function heading = ProperHeading(Heading11,Heading22,Heading33,Heading44):
    | function heading = ProperHeading(Heading11,Heading22,Heading33,Heading44)
    | % This function finds the two headings that match, giving the actual
    | % heading to the pinger
    | 
    | differences = zeros(4,4);
    | 
    | Headings = zeros(1,4);
    | 
    | Headings(1) = Heading11;
    | Headings(2) = Heading22;
    | Headings(3) = Heading33;
    | Headings(4) = Heading44;
    | 
    | for i = 1:4
    |     for j = 1:4
    |         differences(i,j) = abs(Headings(i) - Headings(j));
    |     end
    | end
    | 
    | index = 1;
    | min_dif = 1000;
    | for i = 1:2
    |     for j = 3:4
    |         if(i ~= j)
    |             if(differences(i,j) < min_dif)
    |                 min_dif = differences(i,j);
    |                 index = i;
    |             end
    |         end
    |     end
    | end
    | 
    | if(min_dif < 5)
    |     heading = Headings(index);
    | else
    |     heading = -1;
    | end
    | 
    | return
  function value  = Integrate(r,yaw1,deltaT):
    | function value  = Integrate(r,yaw1,deltaT)
    | % This function performs simple integration
    | 
    | value = r*deltaT + yaw1;
    | 
    | return
  function [Y1,P1,R1] = Integrate3(Yr,Pr,Rr,OY,OP,OR,deltaT):
    | function [Y1,P1,R1] = Integrate3(Yr,Pr,Rr,OY,OP,OR,deltaT)
    | % This function calculates the euler angles using an IMU approach
    | 
    | Y1 = Yr*deltaT + OY;
    | P1 = Pr*deltaT + OP;
    | R1 = Rr*deltaT + OR;
    | 
    | return
  function delta1 = CheckDeltaT(delta):
    | function delta1 = CheckDeltaT(delta)
    | % Make sure deltaT isn't zero breaking everything
    | 
    | if(delta < 0.1)
    |     delta1 = 0.01;
    | else
    |     delta1 = delta/1000;
    | end
    | 
    | return
  function [R_Acc,P_Acc,Y_Acc] = GoToEarthCFrame(RAccB,PAccB,YAccB,y,p,r):
    | function [R_Acc,P_Acc,Y_Acc] = GoToEarthCFrame(RAccB,PAccB,YAccB,y,p,r)
    | % This function uses a rotation matrix to put the accelerations on the
    | % earth based axis using the assumption that the yaw is zero. This gives
    | % the roll and pitch an effect on the accelerations so the strafe thruster
    | % maintains its position in the xy-plane
    | 
    | Accel = zeros(3,1);
    | 
    | yaw = y*pi()/180;
    | pitch = p*pi()/180;
    | roll = r*pi()/180;
    | AccelB = [RAccB;PAccB;YAccB];
    | 
    | % Rotation matrix
    | M = [cos(yaw)*cos(pitch) sin(yaw)*cos(pitch) -sin(pitch);...
    |     cos(yaw)*sin(pitch)*sin(roll)-sin(yaw)*cos(roll) sin(yaw)*sin(pitch)*sin(roll)+cos(yaw)*cos(roll) cos(pitch)*sin(roll);...
    |     cos(yaw)*sin(pitch)*cos(roll)+sin(yaw)*sin(roll) sin(yaw)*sin(roll)*cos(pitch)-cos(yaw)*sin(roll) cos(pitch)*cos(roll)];
    | 
    | Accel = M'*AccelB;
    | 
    | R_Acc = Accel(1);
    | P_Acc = Accel(2);
    | Y_Acc = Accel(3);
    | 
    | return
  function r  = combinevalues(r_m,r1,e1,e2):
    | function r  = combinevalues(r_m,r1,e1,e2)
    | % This function combines information from two sources
    | 
    | x1 = 1 - e1/(e1 + e2);
    | x2 = 1 - e2/(e1 + e2);
    | 
    | r = x1*r_m + x2*r1;
    | 
    | return
  function r  = AUV_Yaw_Model(L1,R1,r_0,deltaT):
    | function r  = AUV_Yaw_Model(L1,R1,r_0,deltaT)
    | % This uses a math model of the auv to calculate the yaw rate and yaw of
    | % the AUV
    | 
    | k = 3.0;
    | 
    | T = L1 - R1;
    | 
    | r_max = 0.0012*T^2 + 0.6913*T + 0.8157;
    | t_max = 0.0006*T^2 + 0.0865*T + 5.6421;
    | 
    | r = k*((r_max-r_0)/t_max)*deltaT + r_0;
    | 
    | if(abs(r_0) < 1.2 && abs(T) < 5)
    |     r = 0;
    | end
    | 
    | return
